simulink model "test_mashinka_mapp_4"  (R2020b)
settings: Solver=ode45  StartTime=0.0  StopTime=20000  RelTol=1e-3  EnableMultiTasking=on
undefined symbols (not defined in the file): CMD_ci_Re_9, CMD_fb, CMD_Firprg_0, CMD_Firprg_1, CMD_gain, CMD_ind_mult, CMD_ind_mult_1, CMD_ind_mult_2, CMD_ind_mult_3, CMD_ind_mult_4, CMD_ind_vol, CMD_ind_vol_1, CMD_ind_vol_2, CMD_ind_vol_3, CMD_ind_vol_4, CMD_nl, CMD_param_0, CMD_pedal, CMD_reset, CMD_shape_0, CMD_step_down, CMD_step_up, ind_mult_0, ind_mult_1, ind_mult_2, ind_mult_3, ind_mult_4, ind_mult_multiplier, num_harm_0, num_pts0, num_str0, num_str1, Res, rom_length
libraries: xbsIndex_r4 x2299
(part 1 of 11)
settings Model: Creator=Dima  LastModifiedBy=Dima
settings DataIOCC: LimitDataPoints=on  SaveFormat=Array  ReturnWorkspaceOutputs=off
settings OptimizationCC: ExpressionDepthLimit=2147483647  LifeSpan=inf
settings DebuggingCC: SolverPrmCheckMsg=warning  StateNameClashWarn=warning  SFUnexpectedBacktrackingDiag=warning  SFNoUnconditionalDefaultTransitionDiag=warning  SFExecutionAtInitializationDiag=none  ArithmeticOperatorsInVariantConditions=warning
settings HardwareCC: ProdBitPerPointer=32  ProdBitPerSizeT=32  ProdBitPerPtrDiffT=32  ProdLargestAtomicFloat=None  ProdIntDivRoundTo=Undefined  ProdEndianess=Unspecified  ProdWordSize=32  ProdHWDeviceType=32-bit Generic
settings ModelReferenceCC: PropagateSignalLabelsOutOfModel=off
settings SFSimCC: SimUseLocalCustomCode=off  CustomCodeUndefinedFunction=UseInterfaceOnly
settings RTWCC: RTWUseLocalCustomCode=off
settings CodeAppCC: StateflowObjectComments=on
settings GRTTargetCC: TargetLangStandard=C89/C90 (ANSI)
settings ConfigComp: CovMetricSettings=dw  CovSaveCumulativeToWorkspaceVar=on  CovSaveSingleToWorkspaceVar=on  CovExternalEMLEnable=off

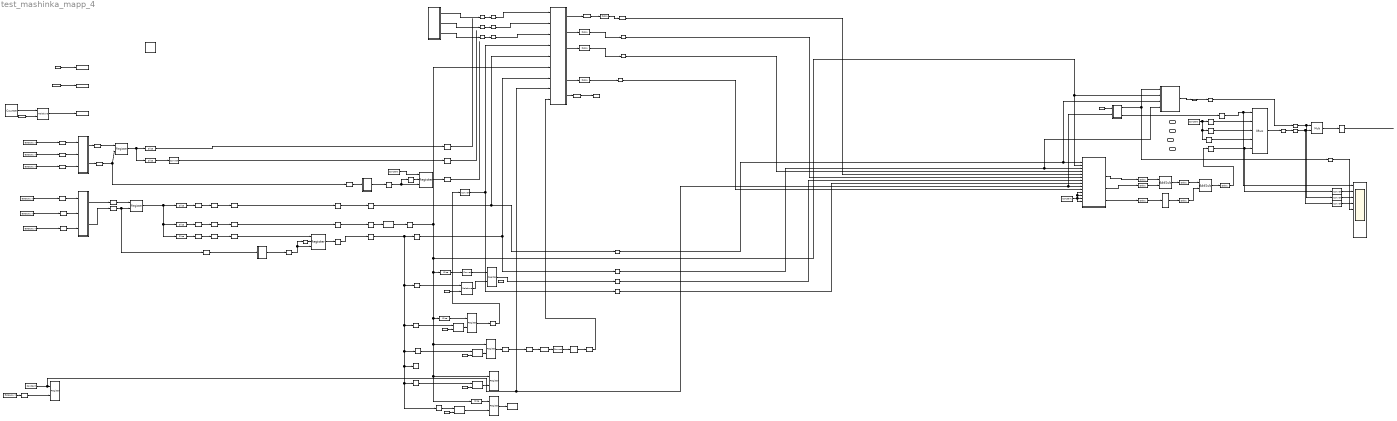
== system test_mashinka_mapp_4 ==
  note: float
  note: prg_en
  note: FIR addr
  force_str36 : Inport
  force_str37 : Inport  Port=2
  force_str38 : Inport  Port=3
  force_str39 : Inport  Port=4
  " System Generator" : xbsIndex_r4/ System Generator  Tag=genX  xilinxfamily=virtexuplus  part=xcvu9p  speed=-2L-e  package=flga2104  synthesis_tool=Vivado  clock_wrapper=Clock Enables  directory=D:/MATLAB_18_prj/Netlist  proj_type=Vivado  Synth_file=Vivado Synthesis Defaults  Impl_file=Vivado Implementation Defaults  testbench=off  simulink_period=1  sysclk_period=10  dcm_input_clock_period=10  incr_netlist=off  trim_vbits=Everywhere in SubSystem  dbl_ovrd=According to Block Masks  core_generation=According to Block Masks  run_coregen=off  deprecated_control=off  eval_field=0  block_type=sysgen
  AddSub4 : xbsIndex_r4/AddSub  mode=Addition  use_carryin=off  use_carryout=off  en=off  latency=8  precision=Full  arith_type=Unsigned  n_bits=16  bin_pt=14  quantization=Truncate  overflow=Wrap  use_behavioral_HDL=off  hw_selection=DSP48  pipelined=on  dbl_ovrd=off  block_type=addsub
  AddSub5 : xbsIndex_r4/AddSub  mode=Addition  use_carryin=off  use_carryout=off  en=off  latency=8  precision=Full  arith_type=Unsigned  n_bits=16  bin_pt=14  quantization=Truncate  overflow=Wrap  use_behavioral_HDL=off  hw_selection=DSP48  pipelined=on  dbl_ovrd=off  block_type=addsub
  CMD_fb : xbsIndex_r4/Constant  const=CMD_fb  gui_display_data_type=Fixed-point  arith_type=Unsigned  n_bits=8  bin_pt=0  preci_type=Single  exp_width=8  frac_width=24  explicit_period=on  period=1  equ=P=C  opselect=C  inp2=PCIN>>17  opr=+  inp1=P  carry=CIN  dbl_ovrd=off  block_type=constant
      settings: block_version=VER_STRING_GOES_HERE
  CMD_gain : xbsIndex_r4/Constant  const=CMD_gain  gui_display_data_type=Fixed-point  arith_type=Unsigned  n_bits=8  bin_pt=0  preci_type=Single  exp_width=8  frac_width=24  explicit_period=on  period=1  equ=P=C  opselect=C  inp2=PCIN>>17  opr=+  inp1=P  carry=CIN  dbl_ovrd=off  block_type=constant
      settings: block_version=VER_STRING_GOES_HERE
  CMD_nl : xbsIndex_r4/Constant  const=CMD_nl  gui_display_data_type=Fixed-point  arith_type=Unsigned  n_bits=8  bin_pt=0  preci_type=Single  exp_width=8  frac_width=24  explicit_period=on  period=1  equ=P=C  opselect=C  inp2=PCIN>>17  opr=+  inp1=P  carry=CIN  dbl_ovrd=off  block_type=constant
      settings: block_version=VER_STRING_GOES_HERE
  CMD_pedal : xbsIndex_r4/Constant  const=CMD_pedal  gui_display_data_type=Fixed-point  arith_type=Unsigned  n_bits=8  bin_pt=0  preci_type=Single  exp_width=8  frac_width=24  explicit_period=on  period=1  equ=P=C  opselect=C  inp2=PCIN>>17  opr=+  inp1=P  carry=CIN  dbl_ovrd=off  block_type=constant
      settings: block_version=VER_STRING_GOES_HERE
  CMD_reset : xbsIndex_r4/Constant  const=CMD_reset  gui_display_data_type=Fixed-point  arith_type=Unsigned  n_bits=8  bin_pt=0  preci_type=Single  exp_width=8  frac_width=24  explicit_period=on  period=1  equ=P=C  opselect=C  inp2=PCIN>>17  opr=+  inp1=P  carry=CIN  dbl_ovrd=off  block_type=constant
      settings: block_version=VER_STRING_GOES_HERE
  Constant : xbsIndex_r4/Constant  const=1  gui_display_data_type=Boolean  arith_type=Boolean  n_bits=16  bin_pt=14  preci_type=Single  exp_width=8  frac_width=24  explicit_period=on  period=1  equ=P=C  opselect=C  inp2=PCIN>>17  opr=+  inp1=P  carry=CIN  dbl_ovrd=off  block_type=constant
  Constant1 : xbsIndex_r4/Constant  const=0  gui_display_data_type=Floating-point  arith_type=Floating-point  n_bits=16  bin_pt=14  preci_type=Single  exp_width=8  frac_width=24  explicit_period=on  period=1  equ=P=C  opselect=C  inp2=PCIN>>17  opr=+  inp1=P  carry=CIN  dbl_ovrd=off  block_type=constant
  Constant2 : xbsIndex_r4/Constant  const=234 - 128 + 19  gui_display_data_type=Fixed-point  arith_type=Unsigned  n_bits=12  bin_pt=0  preci_type=Single  exp_width=8  frac_width=24  explicit_period=off  period=1  equ=P=C  opselect=C  inp2=PCIN>>17  opr=+  inp1=P  carry=CIN  dbl_ovrd=off  block_type=constant
      settings: block_version=VER_STRING_GOES_HERE
  Constant3 : xbsIndex_r4/Constant  const=1  gui_display_data_type=Boolean  arith_type=Boolean  n_bits=16  bin_pt=14  preci_type=Single  exp_width=8  frac_width=24  explicit_period=on  period=1  equ=P=C  opselect=C  inp2=PCIN>>17  opr=+  inp1=P  carry=CIN  dbl_ovrd=off  block_type=constant
  Constant87 : xbsIndex_r4/Constant  const=0  gui_display_data_type=Floating-point  arith_type=Floating-point  n_bits=16  bin_pt=14  preci_type=Single  exp_width=8  frac_width=24  explicit_period=on  period=1  equ=P=C  opselect=C  inp2=PCIN>>17  opr=+  inp1=P  carry=CIN  dbl_ovrd=off  block_type=constant
  Convert1 : xbsIndex_r4/Convert  gui_display_data_type=Floating-point  arith_type=Floating-point  n_bits=16  bin_pt=14  float_type=Single  exp_bits=8  fraction_bits=24  quantization=Truncate  overflow=Wrap  en=off  latency=0  pipeline=off  dbl_ovrd=off  block_type=convert
  Convert12 : xbsIndex_r4/Convert  gui_display_data_type=Boolean  arith_type=Boolean  n_bits=16  bin_pt=14  float_type=Single  exp_bits=8  fraction_bits=24  quantization=Truncate  overflow=Wrap  en=off  latency=0  pipeline=off  dbl_ovrd=off  block_type=convert
  Convert2 : xbsIndex_r4/Convert  gui_display_data_type=Floating-point  arith_type=Floating-point  n_bits=16  bin_pt=14  float_type=Single  exp_bits=8  fraction_bits=24  quantization=Truncate  overflow=Wrap  en=off  latency=0  pipeline=off  dbl_ovrd=off  block_type=convert
  Convert3 : xbsIndex_r4/Convert  gui_display_data_type=Floating-point  arith_type=Floating-point  n_bits=16  bin_pt=14  float_type=Single  exp_bits=8  fraction_bits=24  quantization=Truncate  overflow=Wrap  en=off  latency=0  pipeline=off  dbl_ovrd=off  block_type=convert
  Convert6 : xbsIndex_r4/Convert  gui_display_data_type=Fixed-point  arith_type=Unsigned  n_bits=7  bin_pt=0  float_type=Single  exp_bits=8  fraction_bits=24  quantization=Truncate  overflow=Wrap  en=off  latency=0  pipeline=off  dbl_ovrd=off  block_type=convert
  Convert7 : xbsIndex_r4/Convert  gui_display_data_type=Floating-point  arith_type=Floating-point  n_bits=48  bin_pt=0  float_type=Single  exp_bits=8  fraction_bits=24  quantization="Round  (unbiased: +/- Inf)"  overflow=Saturate  en=off  latency=6  pipeline=off  dbl_ovrd=off  block_type=convert
  Convert8 : xbsIndex_r4/Convert  gui_display_data_type=Fixed-point  arith_type=Unsigned  n_bits=7  bin_pt=0  float_type=Single  exp_bits=8  fraction_bits=24  quantization=Truncate  overflow=Wrap  en=off  latency=0  pipeline=off  dbl_ovrd=off  block_type=convert
  Count2 : Subsystem
  Counter : xbsIndex_r4/Counter  cnt_type=Free Running  cnt_to=Inf  operation=Up  start_count=0  cnt_by_val=1  arith_type=Unsigned  n_bits=20  bin_pt=0  load_pin=off  rst=off  en=off  explicit_period=on  period=1  use_behavioral_HDL=off  implementation=Fabric  dbl_ovrd=off  block_type=counter
  Delay1 : xbsIndex_r4/Delay  rst=off  infoeditControl=Selection of Reset will increase slice count due to use of real FFs and instead of SRLs  en=off  latency=13  reg_retiming=on  dbl_ovrd=off  block_type=delay
      settings: xl_area=[16 32 0 0 0 0 0]  block_version=VER_STRING_GOES_HERE
  Delay{6..9,12..16,18,22,26,30,42,50,54,62,71,83,85..91,127} (27 alike) : xbsIndex_r4/Delay  rst=off  infoeditControl=Selection of Reset will increase slice count due to use of real FFs and instead of SRLs  en=off  latency=1  reg_retiming=on  dbl_ovrd=off  block_type=delay
      Delay12 settings: xl_area=[16 32 0 0 0 0 0]  block_version=VER_STRING_GOES_HERE
      Delay127 settings: xl_area=[2 4 0 4 0 0 0]  block_version=8.2-EVAL
      Delay13 settings: xl_area=[16 32 0 0 0 0 0]  block_version=VER_STRING_GOES_HERE
      Delay14 settings: xl_area=[16 32 0 0 0 0 0]  block_version=VER_STRING_GOES_HERE
      Delay15 settings: xl_area=[16 32 0 0 0 0 0]  block_version=VER_STRING_GOES_HERE
      Delay16 settings: xl_area=[16 32 0 0 0 0 0]  block_version=VER_STRING_GOES_HERE
      Delay18 settings: xl_area=[16 32 0 0 0 0 0]  block_version=VER_STRING_GOES_HERE
      Delay22 settings: xl_area=[2 4 0 4 0 0 0]  block_version=8.2-EVAL
      Delay26 settings: xl_area=[16 32 0 0 0 0 0]  block_version=VER_STRING_GOES_HERE
      Delay30 settings: xl_area=[2 4 0 4 0 0 0]  block_version=8.2-EVAL
      Delay42 settings: xl_area=[16 32 0 0 0 0 0]  block_version=VER_STRING_GOES_HERE
      Delay50 settings: xl_area=[16 32 0 0 0 0 0]  block_version=VER_STRING_GOES_HERE
      Delay54 settings: xl_area=[16 32 0 0 0 0 0]  block_version=VER_STRING_GOES_HERE
      Delay6 settings: xl_area=[16 32 0 0 0 0 0]  block_version=VER_STRING_GOES_HERE
      Delay62 settings: xl_area=[16 32 0 0 0 0 0]  block_version=VER_STRING_GOES_HERE
      Delay7 settings: xl_area=[16 32 0 0 0 0 0]  block_version=VER_STRING_GOES_HERE
      Delay71 settings: xl_area=[2 4 0 4 0 0 0]  block_version=8.2-EVAL
      Delay8 settings: xl_area=[16 32 0 0 0 0 0]  block_version=VER_STRING_GOES_HERE
      Delay83 settings: xl_area=[16 32 0 0 0 0 0]  block_version=VER_STRING_GOES_HERE
      Delay85 settings: xl_area=[16 32 0 0 0 0 0]  block_version=VER_STRING_GOES_HERE
      Delay86 settings: xl_area=[16 32 0 0 0 0 0]  block_version=VER_STRING_GOES_HERE
      Delay87 settings: xl_area=[16 32 0 0 0 0 0]  block_version=VER_STRING_GOES_HERE
      Delay88 settings: xl_area=[16 32 0 0 0 0 0]  block_version=VER_STRING_GOES_HERE
      Delay89 settings: xl_area=[16 32 0 0 0 0 0]  block_version=VER_STRING_GOES_HERE
      Delay9 settings: xl_area=[16 32 0 0 0 0 0]  block_version=VER_STRING_GOES_HERE
      Delay90 settings: xl_area=[16 32 0 0 0 0 0]  block_version=VER_STRING_GOES_HERE
      Delay91 settings: xl_area=[16 32 0 0 0 0 0]  block_version=VER_STRING_GOES_HERE
  Delay23 : xbsIndex_r4/Delay  rst=off  infoeditControl=Selection of Reset will increase slice count due to use of real FFs and instead of SRLs  en=off  latency=7  reg_retiming=on  dbl_ovrd=off  block_type=delay
      settings: xl_area=[16 32 0 0 0 0 0]  block_version=VER_STRING_GOES_HERE
  Delay25 : xbsIndex_r4/Delay  rst=off  infoeditControl=Selection of Reset will increase slice count due to use of real FFs and instead of SRLs  en=off  latency=4  reg_retiming=on  dbl_ovrd=off  block_type=delay
      settings: xl_area=[16 32 0 0 0 0 0]  block_version=VER_STRING_GOES_HERE
  Delay27 : xbsIndex_r4/Delay  rst=off  infoeditControl=Selection of Reset will increase slice count due to use of real FFs and instead of SRLs  en=off  latency=4  reg_retiming=on  dbl_ovrd=off  block_type=delay
      settings: xl_area=[16 32 0 0 0 0 0]  block_version=VER_STRING_GOES_HERE
  Delay28 : xbsIndex_r4/Delay  rst=off  infoeditControl=Selection of Reset will increase slice count due to use of real FFs and instead of SRLs  en=off  latency=40  reg_retiming=on  dbl_ovrd=off  block_type=delay
      settings: xl_area=[16 32 0 0 0 0 0]  block_version=VER_STRING_GOES_HERE
  Delay29 : xbsIndex_r4/Delay  rst=off  infoeditControl=Selection of Reset will increase slice count due to use of real FFs and instead of SRLs  en=off  latency=14  reg_retiming=off  dbl_ovrd=off  block_type=delay
  Delay31 : xbsIndex_r4/Delay  rst=off  infoeditControl=Selection of Reset will increase slice count due to use of real FFs and instead of SRLs  en=off  latency=11  reg_retiming=on  dbl_ovrd=off  block_type=delay
      settings: xl_area=[2 4 0 4 0 0 0]  block_version=8.2-EVAL
  Delay32 : xbsIndex_r4/Delay  rst=off  infoeditControl=Selection of Reset will increase slice count due to use of real FFs and instead of SRLs  en=off  latency=11  reg_retiming=on  dbl_ovrd=off  block_type=delay
      settings: xl_area=[2 4 0 4 0 0 0]  block_version=8.2-EVAL
  Delay{35..41,43..46,52,78..82} (17 alike) : xbsIndex_r4/Delay  rst=off  infoeditControl=Selection of Reset will increase slice count due to use of real FFs and instead of SRLs  en=off  latency=1  reg_retiming=off  dbl_ovrd=off  block_type=delay
      settings: block_version=9.1.01-EVAL
  Delay84 : xbsIndex_r4/Delay  rst=off  infoeditControl=Selection of Reset will increase slice count due to use of real FFs and instead of SRLs  en=off  latency=10  reg_retiming=on  dbl_ovrd=off  block_type=delay
      settings: xl_area=[16 32 0 0 0 0 0]  block_version=VER_STRING_GOES_HERE
  Gateway Out3 : xbsIndex_r4/Gateway Out  inherit_from_input=off  hdl_port=off  rows=1  columns=1  UseAsDAC=off  DACChannel='1'  interface=None  automatic_assignment=on  address_offset=hex2dec('00')  intf_name=''  intf_description=''  timing_constraint=None  locs_specified=off  LOCs={}  io_standard={}  block_type=gatewayout
  Gateway Out4 : xbsIndex_r4/Gateway Out  inherit_from_input=off  hdl_port=off  rows=1  columns=1  UseAsDAC=off  DACChannel='1'  interface=None  automatic_assignment=on  address_offset=hex2dec('00')  intf_name=''  intf_description=''  timing_constraint=None  locs_specified=off  LOCs={}  io_standard={}  block_type=gatewayout
  Gateway Out6 : xbsIndex_r4/Gateway Out  inherit_from_input=off  hdl_port=off  rows=1  columns=1  UseAsDAC=off  DACChannel='1'  interface=None  automatic_assignment=on  address_offset=hex2dec('00')  intf_name=''  intf_description=''  timing_constraint=None  locs_specified=off  LOCs={}  io_standard={}  block_type=gatewayout
  Mid_Graph1 : Subsystem
  Mult10 : xbsIndex_r4/Mult  precision=Full  arith_type="Signed  (2's comp)"  n_bits=16  bin_pt=14  quantization=Truncate  overflow=Wrap  en=off  latency=6  use_behavioral_HDL=off  opt=Speed  use_embedded=on  optimum_pipeline=off  pipeline=on  dbl_ovrd=off  use_rpm=on  placement_style=Triangular  block_type=mult
  Mux10 : xbsIndex_r4/Mux  inputs=4  en=off  latency=1  precision=Full  arith_type=Unsigned  n_bits=16  bin_pt=14  quantization=Truncate  overflow=Wrap  dbl_ovrd=off  block_type=mux
  RSlice12 : xbsIndex_r4/Slice  nbits=32  boolean_output=off  mode=Lower Bit Location + Width  bit1=0  base1=MSB of Input  bit0=8  base0=LSB of Input  dbl_ovrd=off  block_type=slice
      settings: block_version=VER_STRING_GOES_HERE
  RSlice13 : xbsIndex_r4/Slice  nbits=10  boolean_output=off  mode=Lower Bit Location + Width  bit1=0  base1=MSB of Input  bit0=40  base0=LSB of Input  dbl_ovrd=off  block_type=slice
      settings: block_version=VER_STRING_GOES_HERE
  RSlice14 : xbsIndex_r4/Slice  nbits=8  boolean_output=off  mode=Lower Bit Location + Width  bit1=0  base1=MSB of Input  bit0=0  base0=LSB of Input  dbl_ovrd=off  block_type=slice
      settings: block_version=VER_STRING_GOES_HERE
  RSlice4 : xbsIndex_r4/Slice  nbits=1  boolean_output=off  mode=Lower Bit Location + Width  bit1=0  base1=MSB of Input  bit0=0  base0=LSB of Input  dbl_ovrd=off  block_type=slice
      settings: block_version=VER_STRING_GOES_HERE
  RSlice7 : xbsIndex_r4/Slice  nbits=7  boolean_output=off  mode=Lower Bit Location + Width  bit1=0  base1=MSB of Input  bit0=0  base0=LSB of Input  dbl_ovrd=off  block_type=slice
      settings: block_version=VER_STRING_GOES_HERE
  RSlice8 : xbsIndex_r4/Slice  nbits=4  boolean_output=off  mode=Lower Bit Location + Width  bit1=0  base1=MSB of Input  bit0=0  base0=LSB of Input  dbl_ovrd=off  block_type=slice
      settings: block_version=VER_STRING_GOES_HERE
  Reciever16 : Subsystem
  Reciever50 : Subsystem
  Register{1,5,10..13,17..19,23..24,27..29,41,78..86,460,462..464} (28 alike) : xbsIndex_r4/Register  init=0  rst=off  en=off  dbl_ovrd=off  block_type=register
  Register14 : xbsIndex_r4/Register  init=0  rst=on  en=on  dbl_ovrd=off  block_type=register
      settings: block_version=8.2-EVAL
  Register{38,40,43,47..48,52,61,183} (8 alike) : xbsIndex_r4/Register  init=0  rst=off  en=on  dbl_ovrd=off  block_type=register
      Register40 settings: block_version=8.2-EVAL
      Register61 settings: block_version=8.2-EVAL
  Register4 : xbsIndex_r4/Register  init=0  rst=on  en=on  dbl_ovrd=off  block_type=register
      settings: block_version=8.2-EVAL
  Reinterpret10 : xbsIndex_r4/Reinterpret  force_arith_type=on  arith_type=Floating-point  force_bin_pt=on  bin_pt=24  block_type=reinterpret
  Reinterpret3 : xbsIndex_r4/Reinterpret  force_arith_type=on  arith_type="Signed  (2's comp)"  force_bin_pt=on  bin_pt=0  block_type=reinterpret
  Reinterpret4 : xbsIndex_r4/Reinterpret  force_arith_type=on  arith_type=Unsigned  force_bin_pt=on  bin_pt=0  block_type=reinterpret
  Relational{2..4,6,10,14} (6 alike) : xbsIndex_r4/Relational  mode=a=b  op_type=Bool  en=off  latency=0  dbl_ovrd=off  block_type=relational
  SIMULATION : Subsystem
  Scope1 : Scope  NumInputPorts=9
  a : xbsIndex_r4/Constant  const=2000  gui_display_data_type=Fixed-point  arith_type=Unsigned  n_bits=20  bin_pt=0  preci_type=Single  exp_width=8  frac_width=24  explicit_period=on  period=1  equ=P=C  opselect=C  inp2=PCIN>>17  opr=+  inp1=P  carry=CIN  dbl_ovrd=off  block_type=constant
      settings: block_version=VER_STRING_GOES_HERE
  a1 : xbsIndex_r4/Constant  const=1  gui_display_data_type=Fixed-point  arith_type=Unsigned  n_bits=10  bin_pt=0  preci_type=Single  exp_width=8  frac_width=24  explicit_period=on  period=1  equ=P=C  opselect=C  inp2=PCIN>>17  opr=+  inp1=P  carry=CIN  dbl_ovrd=off  block_type=constant
      settings: block_version=VER_STRING_GOES_HERE
  a2 : xbsIndex_r4/Constant  const=10000  gui_display_data_type=Fixed-point  arith_type=Unsigned  n_bits=32  bin_pt=0  preci_type=Single  exp_width=8  frac_width=24  explicit_period=on  period=1  equ=P=C  opselect=C  inp2=PCIN>>17  opr=+  inp1=P  carry=CIN  dbl_ovrd=off  block_type=constant
      settings: block_version=VER_STRING_GOES_HERE
  ci_re_9 : Subsystem
  clk_16_in : xbsIndex_r4/Gateway In  gui_display_data_type=Fixed-point  arith_type=Unsigned  n_bits=1  bin_pt=0  preci_type=Single  exp_width=8  frac_width=24  rows=1  columns=1  quantization="Round  (unbiased: +/- Inf)"  overflow=Saturate  period=1  UseAsADC=off  ADCChannel='1'  interface=None  automatic_assignment=on  address_offset=hex2dec('00')  intf_name=''  intf_description=''  default_value=0  timing_constraint=None  locs_specified=off  LOCs={'AE32'}  io_standard={}  inherit_from_input=off  hdl_port=on  dbl_ovrd=off  block_type=gatewayin
      settings: block_version=11.4
  clk_50_in : xbsIndex_r4/Gateway In  gui_display_data_type=Fixed-point  arith_type=Unsigned  n_bits=1  bin_pt=0  preci_type=Single  exp_width=8  frac_width=24  rows=1  columns=1  quantization="Round  (unbiased: +/- Inf)"  overflow=Saturate  period=1  UseAsADC=off  ADCChannel='1'  interface=None  automatic_assignment=on  address_offset=hex2dec('00')  intf_name=''  intf_description=''  default_value=0  timing_constraint=None  locs_specified=off  LOCs={'AE32'}  io_standard={}  inherit_from_input=off  hdl_port=on  dbl_ovrd=off  block_type=gatewayin
      settings: block_version=11.4
  curr{14..17,24..25} (6 alike) : xbsIndex_r4/Delay  rst=off  infoeditControl=Selection of Reset will increase slice count due to use of real FFs and instead of SRLs  en=off  latency=1  reg_retiming=on  dbl_ovrd=off  block_type=delay
      settings: xl_area=[16 32 0 0 0 0 0]  block_version=VER_STRING_GOES_HERE
  curr18 : xbsIndex_r4/Delay  rst=off  infoeditControl=Selection of Reset will increase slice count due to use of real FFs and instead of SRLs  en=off  latency=8  reg_retiming=on  dbl_ovrd=off  block_type=delay
      settings: xl_area=[16 32 0 0 0 0 0]  block_version=VER_STRING_GOES_HERE
  en1 : Subsystem
  en2 : Subsystem
  frm_16_in : xbsIndex_r4/Gateway In  gui_display_data_type=Fixed-point  arith_type=Unsigned  n_bits=1  bin_pt=0  preci_type=Single  exp_width=8  frac_width=24  rows=1  columns=1  quantization="Round  (unbiased: +/- Inf)"  overflow=Saturate  period=1  UseAsADC=off  ADCChannel='1'  interface=None  automatic_assignment=on  address_offset=hex2dec('00')  intf_name=''  intf_description=''  default_value=0  timing_constraint=None  locs_specified=off  LOCs={'AH34'}  io_standard={}  inherit_from_input=off  hdl_port=on  dbl_ovrd=off  block_type=gatewayin
      settings: block_version=11.4
  frm_50_in : xbsIndex_r4/Gateway In  gui_display_data_type=Fixed-point  arith_type=Unsigned  n_bits=1  bin_pt=0  preci_type=Single  exp_width=8  frac_width=24  rows=1  columns=1  quantization="Round  (unbiased: +/- Inf)"  overflow=Saturate  period=1  UseAsADC=off  ADCChannel='1'  interface=None  automatic_assignment=on  address_offset=hex2dec('00')  intf_name=''  intf_description=''  default_value=0  timing_constraint=None  locs_specified=off  LOCs={'AH34'}  io_standard={}  inherit_from_input=off  hdl_port=on  dbl_ovrd=off  block_type=gatewayin
      settings: block_version=11.4
  mashinka_0 : Subsystem  mask{nota_0_0=44, nota_0_1=45, nota_0_2=45, nota_0_3=45, addr_str_0_0=512, addr_str_0_1=413, addr_str_0_2=446, addr_str_0_3=479, prm0=CMD_param_0, shape0=CMD_shape_0}
  n1 : xbsIndex_r4/Slice  nbits=7  boolean_output=off  mode=Lower Bit Location + Width  bit1=0  base1=MSB of Input  bit0=0  base0=LSB of Input  dbl_ovrd=off  block_type=slice
      settings: block_version=VER_STRING_GOES_HERE
  pedal : xbsIndex_r4/Constant  const=70  gui_display_data_type=Fixed-point  arith_type=Unsigned  n_bits=7  bin_pt=0  preci_type=Single  exp_width=8  frac_width=24  explicit_period=on  period=1  equ=P=C  opselect=C  inp2=PCIN>>17  opr=+  inp1=P  carry=CIN  dbl_ovrd=off  block_type=constant
      settings: block_version=VER_STRING_GOES_HERE
  sdat_16_in : xbsIndex_r4/Gateway In  gui_display_data_type=Fixed-point  arith_type=Unsigned  n_bits=1  bin_pt=0  preci_type=Single  exp_width=8  frac_width=24  rows=1  columns=1  quantization="Round  (unbiased: +/- Inf)"  overflow=Saturate  period=1  UseAsADC=off  ADCChannel='1'  interface=None  automatic_assignment=on  address_offset=hex2dec('00')  intf_name=''  intf_description=''  default_value=0  timing_constraint=None  locs_specified=off  LOCs={'AJ32'}  io_standard={}  inherit_from_input=off  hdl_port=on  dbl_ovrd=off  block_type=gatewayin
      settings: block_version=11.4
  sdat_50_in : xbsIndex_r4/Gateway In  gui_display_data_type=Fixed-point  arith_type=Unsigned  n_bits=1  bin_pt=0  preci_type=Single  exp_width=8  frac_width=24  rows=1  columns=1  quantization="Round  (unbiased: +/- Inf)"  overflow=Saturate  period=1  UseAsADC=off  ADCChannel='1'  interface=None  automatic_assignment=on  address_offset=hex2dec('00')  intf_name=''  intf_description=''  default_value=0  timing_constraint=None  locs_specified=off  LOCs={'AJ32'}  io_standard={}  inherit_from_input=off  hdl_port=on  dbl_ovrd=off  block_type=gatewayin
      settings: block_version=11.4
  start : xbsIndex_r4/Gateway In  gui_display_data_type=Boolean  arith_type=Boolean  n_bits=1  bin_pt=0  preci_type=Single  exp_width=8  frac_width=24  rows=1  columns=1  quantization="Round  (unbiased: +/- Inf)"  overflow=Saturate  period=1  UseAsADC=off  ADCChannel='1'  interface=None  automatic_assignment=on  address_offset=hex2dec('00')  intf_name=''  intf_description=''  default_value=0  timing_constraint=None  locs_specified=off  LOCs={'AH34'}  io_standard={}  inherit_from_input=off  hdl_port=on  dbl_ovrd=off  block_type=gatewayin
      settings: block_version=11.4
  v1 : xbsIndex_r4/Slice  nbits=8  boolean_output=off  mode=Upper Bit Location + Width  bit1=0  base1=MSB of Input  bit0=8  base0=LSB of Input  dbl_ovrd=off  block_type=slice
      settings: block_version=VER_STRING_GOES_HERE
  wires:
  Register4/1 -> Delay9/1
  Delay7/1 -> Reinterpret3/1
  Delay13/1 -> Delay6/1
  Register183/1 -> Register463/1
  RSlice7/1 -> Convert6/1
  Convert6/1 -> Register183/1
  CMD_pedal/1 -> Relational14/2
  Relational14/1 -> Register183/2
  Convert12/1 -> Mid_Graph1/4(RST), Register464/1
  Delay37/1 -> Register12/1
  Delay39/1 -> Register11/1
  Delay38/1 -> Register10/1
  Delay27/1 -> Register5/1, Register4/3
  Register5/1 -> Register4/2
  Register10/1 -> Delay13/1
  Register12/1 -> Register4/1
  a/1 -> Relational2/2
  Counter/1 -> Relational2/1
  a1/1 -> Gateway Out3/1
  a2/1 -> Gateway Out4/1
  Delay9/1 -> Delay8/1
  Delay12/1 -> Delay7/1
  Delay15/1 -> Mid_Graph1/7(mem_en), Register462/1
  Delay16/1 -> Relational14/1
  Relational2/1 -> Gateway Out6/1
  Register84/1 -> mashinka_0/6(NN)
  Register460/1 -> mashinka_0/1(Addr_param), ci_re_9/3(m_addr)
  Register463/1 -> mashinka_0/7(Pedal)
  Register85/1 -> mashinka_0/4(Addr)
  Delay30/1 -> mashinka_0/5(force)
  Register47/1 -> Register41/1
  CMD_nl/1 -> Relational3/2
  Relational3/1 -> Register47/2
  Delay42/1 -> Relational3/1
  Relational4/1 -> Register48/2
  CMD_fb/1 -> Relational4/2
  Delay50/1 -> Relational4/1
  Register52/1 -> Reinterpret4/1
  Delay54/1 -> Relational6/1
  Relational6/1 -> Register52/2
  CMD_gain/1 -> Relational6/2
  RSlice8/1 -> Register52/1
  Register11/1 -> Delay12/1
  RSlice4/1 -> Register38/1
  Register38/1 -> Delay62/1
  CMD_reset/1 -> Relational10/2
  Relational10/1 -> Register38/2
  Delay26/1 -> Relational10/1
  Delay62/1 -> Convert12/1
  Delay78/1 -> Register13/1, Register61/2
  Delay35/1 -> Register61/1
  RSlice13/1 -> Delay81/1
  Register61/1 -> RSlice14/1, RSlice12/1, RSlice13/1
  sdat_50_in/1 -> Delay80/1
  RSlice12/1 -> Delay82/1
  Delay80/1 -> Reciever50/1(s_dat)
  Delay36/1 -> Delay37/1
  Delay82/1 -> Delay39/1
  Reciever50/2(reset_z1) -> Delay78/1
  Delay79/1 -> Reciever50/2(clk)
  clk_50_in/1 -> Delay79/1
  frm_50_in/1 -> Delay40/1
  Delay40/1 -> Reciever50/3(frm)
  Reciever50/1(Out1) -> Delay35/1
  Delay81/1 -> Delay38/1
  RSlice14/1 -> Delay36/1
  Reinterpret3/1 -> Delay14/1
  Delay41/1 -> Reciever16/3(frm)
  frm_16_in/1 -> Delay41/1
  clk_16_in/1 -> Delay43/1
  sdat_16_in/1 -> Delay44/1
  Reciever16/1(Out1) -> Delay45/1
  Delay44/1 -> Reciever16/1(s_dat)
  Reciever16/2(reset_z1) -> Delay46/1
  Delay45/1 -> Register40/1
  Delay43/1 -> Reciever16/2(clk)
  Register13/1 -> en1/1(In1)
  en1/1(Out1) -> Delay27/1
  n1/1 -> Convert8/1
  Register40/1 -> n1/1, v1/1
  v1/1 -> Register17/1
  Convert8/1 -> Register18/1
  Constant/1 -> Register14/1
  Delay28/1 -> Register14/2
  Delay25/1 -> Register14/3, Delay28/1
  en2/1(Out1) -> Delay25/1
  Register14/1 -> Register19/1
  Register27/1 -> en2/1(In1)
  Delay46/1 -> Register27/1, Register40/2
  start/1 -> Delay52/1
  Delay52/1 -> Register43/2
  Register464/1 -> mashinka_0/8(Reset)
  Register83/1 -> Mid_Graph1/3(mid_en)
  Register82/1 -> Mid_Graph1/2(nota)
  Register81/1 -> Register83/1
  Register80/1 -> Register82/1
  Register79/1 -> Mid_Graph1/1(vol)
  Register78/1 -> Register79/1
  Register28/1 -> Mid_Graph1/9(noise_mult)
  Mid_Graph1/5(nn_fl) -> Delay31/1
  Delay31/1 -> Register86/1
  Mid_Graph1/2(nn) -> Delay32/1
  Delay32/1 -> Register84/1
  Delay29/1 -> Register85/1
  Mid_Graph1/3(addr) -> Delay29/1
  Register86/1 -> mashinka_0/10(nn_fl)
  Register17/1 -> ?
  Register18/1 -> ?
  Register19/1 -> ?
  Reinterpret10/1 -> Convert7/1
  Register29/1 -> Reinterpret10/1
  Convert7/1 -> Register24/1
  Register24/1 -> Register28/1
  Register41/1 -> Register29/1
  Delay22/1 -> Delay23/1
  Mid_Graph1/1(FF_out) -> Delay22/1
  Delay23/1 -> Delay30/1
  Constant3/1 -> Mid_Graph1/8(start), mashinka_0/9(start), Count2/2(start), Register43/1
  Delay6/1 -> Mid_Graph1/5(mem_addr), Register460/1
  Delay14/1 -> Mid_Graph1/6(mem_dat), mashinka_0/2(Dat_param), ci_re_9/2(m_data), RSlice4/1, RSlice8/1, Register48/1, Register47/1, RSlice7/1
  Delay8/1 -> Delay26/1, Delay42/1, Delay54/1, Delay50/1, Delay18/1, Delay16/1, Delay15/1
  Mid_Graph1/6(FF_stuk) -> Delay71/1
  Delay71/1 -> Delay127/1
  Register462/1 -> mashinka_0/3(we_param), ci_re_9/4(m_en)
  SIMULATION/1(vol) -> Register78/1
  SIMULATION/2(nota) -> Register80/1
  SIMULATION/3(en) -> Register81/1
  Constant1/1 -> mashinka_0/13(LASTX2), mashinka_0/14(LASTX3), mashinka_0/11(LASTX0), mashinka_0/12(LASTX1)
  mashinka_0/4(out_3) -> curr16/1
  mashinka_0/3(out_2) -> curr14/1
  curr14/1 -> AddSub5/2
  AddSub4/1 -> curr25/1
  mashinka_0/2(out_1) -> curr17/1
  curr17/1 -> AddSub5/1
  AddSub5/1 -> curr15/1
  curr15/1 -> AddSub4/1
  curr18/1 -> curr24/1
  curr16/1 -> curr18/1
  curr24/1 -> AddSub4/2
  Register23/1 -> Delay83/1
  Register1/1 -> ?
  Delay87/1 -> Mux10/4
  Delay84/1 -> Delay90/1
  Delay88/1 -> Convert1/1, Mux10/5
  Delay91/1 -> Scope1/1, Mux10/1
  Delay89/1 -> Convert2/1, Mult10/1
  Delay86/1 -> Mux10/3
  ci_re_9/1(Out) -> Register23/1
  Mux10/1 -> Delay84/1
  Delay90/1 -> Convert3/1, Mult10/2
  Delay85/1 -> Mux10/2
  Delay83/1 -> Delay89/1
  Count2/3(Out3) -> Delay91/1
  Mult10/1 -> Register1/1
  Constant2/1 -> Count2/1(In1)
  Count2/1(addr) -> Delay1/1, ci_re_9/1(addr)
  curr25/1 -> Delay88/1
  Constant87/1 -> Delay86/1, Delay87/1, Delay85/1
  Convert1/1 -> Scope1/2
  Convert2/1 -> Scope1/3
  Convert3/1 -> Scope1/4
  Delay1/1 -> Scope1/5

== system test_mashinka_mapp_4/Count2 ==
  In1 : Inport
  start : Inport  Port=2
  Constant1 : xbsIndex_r4/Constant  const=1  gui_display_data_type=Fixed-point  arith_type=Boolean  n_bits=5  bin_pt=0  preci_type=Single  exp_width=8  frac_width=24  explicit_period=off  period=1  equ=P=C  opselect=C  inp2=PCIN>>17  opr=+  inp1=P  carry=CIN  dbl_ovrd=off  block_type=constant
      settings: block_version=VER_STRING_GOES_HERE
  Counter1 : xbsIndex_r4/Counter  cnt_type=Free Running  cnt_to=1  operation=Up  start_count=0  cnt_by_val=1  arith_type=Unsigned  n_bits=10  bin_pt=0  load_pin=off  rst=off  en=on  explicit_period=on  period=1  use_behavioral_HDL=off  implementation=Fabric  use_rpm=off  dbl_ovrd=off  block_type=counter
      settings: block_version=8.2.02
  Counter2 : xbsIndex_r4/Counter  cnt_type=Free Running  cnt_to=15  operation=Up  start_count=0  cnt_by_val=1  arith_type=Unsigned  n_bits=9  bin_pt=0  load_pin=off  rst=off  en=on  explicit_period=on  period=1  use_behavioral_HDL=off  implementation=Fabric  use_rpm=off  dbl_ovrd=off  block_type=counter
      settings: block_version=8.2.02
  Delay2 : xbsIndex_r4/Delay  rst=off  infoeditControl=Selection of Reset will increase slice count due to use of real FFs and instead of SRLs  en=off  latency=1  reg_retiming=on  dbl_ovrd=off  block_type=delay
      settings: xl_area=[2 4 0 4 0 0 0]  block_version=8.2-EVAL
  RSlice1 : xbsIndex_r4/Slice  nbits=ceil(log2(2*num_str0))  boolean_output=off  mode=Lower Bit Location + Width  bit1=0  base1=MSB of Input  bit0=6  base0=LSB of Input  dbl_ovrd=off  block_type=slice
      settings: block_version=VER_STRING_GOES_HERE
  RSlice2 : xbsIndex_r4/Slice  nbits=2  boolean_output=off  mode=Upper Bit Location + Width  bit1=0  base1=MSB of Input  bit0=7  base0=LSB of Input  dbl_ovrd=off  block_type=slice
      settings: block_version=VER_STRING_GOES_HERE
  Register6 : xbsIndex_r4/Register  init=0  rst=off  en=on  dbl_ovrd=off  block_type=register
  Relational1 : xbsIndex_r4/Relational  mode=a=b  op_type=Bool  en=off  latency=1  dbl_ovrd=off  block_type=relational
      settings: xl_area=[4 1 0 7 0 0 0]  block_version=VER_STRING_GOES_HERE
  Scope1 : Scope  NumInputPorts=8
  addr : Outport  VectorParamsAs1DForOutWhenUnconnected=off
  Out2 : Outport  Port=2  VectorParamsAs1DForOutWhenUnconnected=off
  Out3 : Outport  Port=3  VectorParamsAs1DForOutWhenUnconnected=off
  wires:
  start/1 -> Delay2/1
  Delay2/1 -> Counter1/1
  Counter2/1 -> Scope1/1, RSlice2/1, RSlice1/1, addr/1
  Counter1/1 -> Relational1/1
  Constant1/1 -> Register6/1
  Relational1/1 -> Register6/2
  Register6/1 -> Counter2/1
  In1/1 -> Relational1/2
  RSlice1/1 -> Out2/1
  RSlice2/1 -> Scope1/2, Out3/1
